simulink model "assignment1_ofmbd"  (R2020b)
settings: Solver=VariableStepAuto  StartTime=0.0  StopTime=100  RelTol=1e-3
values from neighbouring files (symbols this model uses):
  b = 50    [assignment1.mat]
  M1 = 100    [assignment1.mat]
  M2 = 95    [assignment1.mat]
undefined symbols (not defined in the file or in its folder): k1, k12
settings Model: Creator=Shree  LastModifiedBy=Shree

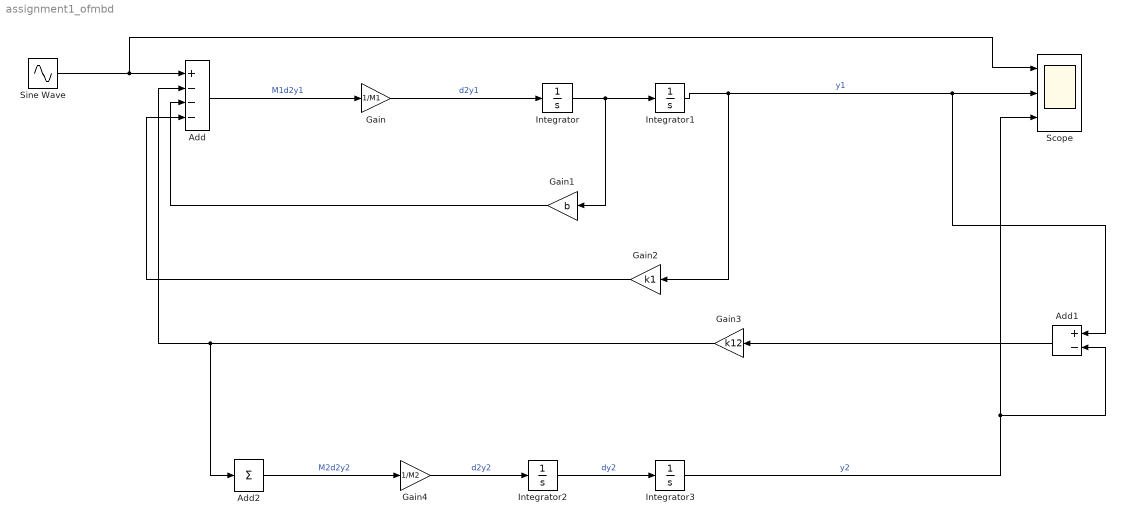
== system assignment1_ofmbd ==
  Add : Sum  Inputs=+---
  Add1 : Sum  Inputs=+-
  Add2 : Sum  Inputs=+
  Gain : Gain  Gain=1/M1
  Gain1 : Gain  Gain=b
  Gain2 : Gain  Gain=k1
  Gain3 : Gain  Gain=k12
  Gain4 : Gain  Gain=1/M2
  Integrator{,1..3} (4 alike) : Integrator
  Scope : Scope  NumInputPorts=3
  Sine Wave : Sin  SampleTime=0
  wires:
  Gain/1 -> Integrator/1  "d2y1"
  Integrator/1 -> Gain1/1, Integrator1/1
  Gain3/1 -> Add2/1, Add/2
  Add2/1 -> Gain4/1  "M2d2y2"
  Gain1/1 -> Add/3
  Gain2/1 -> Add/4
  Integrator2/1 -> Integrator3/1  "dy2"
  Add1/1 -> Gain3/1
  Sine Wave/1 -> Scope/1, Add/1
  Gain4/1 -> Integrator2/1  "d2y2"
  Integrator3/1 -> Scope/3, Add1/2  "y2"
  Integrator1/1 -> Gain2/1, Add1/1, Scope/2  "y1"
  Add/1 -> Gain/1  "M1d2y1"
